simulink model "3-6-3"  (R2022b)
settings: Solver=VariableStepAuto  StartTime=0.0  StopTime=10.0  RelTol=1e-3
settings Model: Creator=Mavara-(Asus)  LastModifiedBy=Mavara-(Asus)

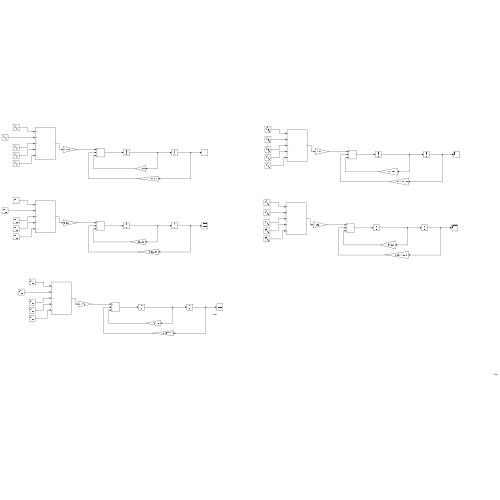
[thumbnail: Simulink's stored preview of the top-level diagram]
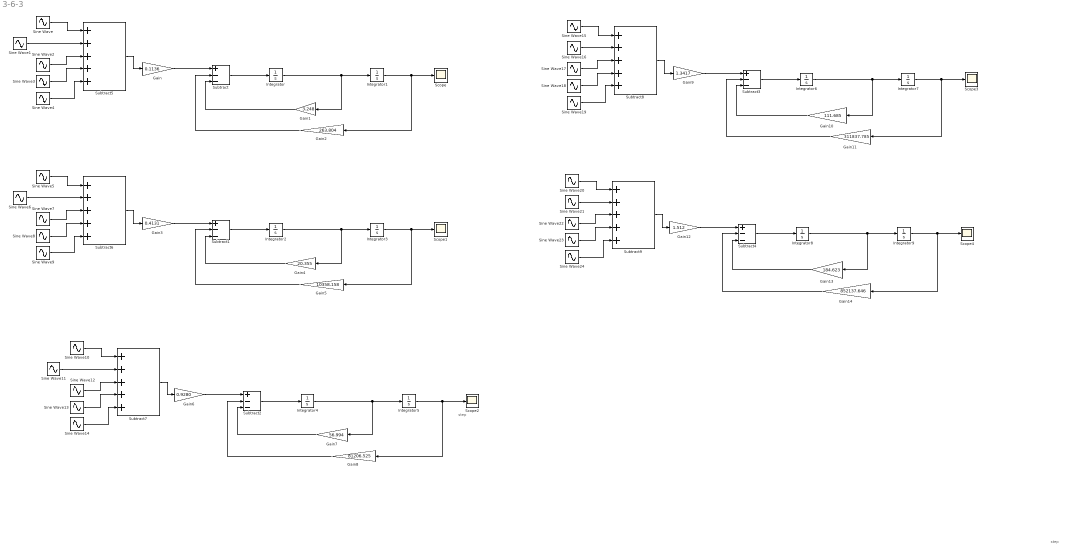
== system 3-6-3 ==
  note: step
  note: step
  Gain : Gain  Gain=0.1136
  Gain1 : Gain  Gain=3.248
  Gain10 : Gain  Gain=111.685
  Gain11 : Gain  Gain=311837.785
  Gain12 : Gain  Gain=1.512
  Gain13 : Gain  Gain=184.623
  Gain14 : Gain  Gain=852137.646
  Gain2 : Gain  Gain=263.804
  Gain3 : Gain  Gain=0.4131
  Gain4 : Gain  Gain=20.355
  Gain5 : Gain  Gain=10358.158
  Gain6 : Gain  Gain=0.9280
  Gain7 : Gain  Gain=56.994
  Gain8 : Gain  Gain=81206.525
  Gain9 : Gain  Gain=1.3417
  Integrator{,1..9} (10 alike) : Integrator
  Scope{,1..4} (5 alike) : Scope
  Sine Wave : Sin  Frequency=16.2338  SampleTime=0
  Sine Wave1 : Sin  Frequency=101.72344  SampleTime=0
  Sine Wave10 : Sin  Frequency=16.2338  SampleTime=0
  Sine Wave11 : Sin  Frequency=101.72344  SampleTime=0
  Sine Wave12 : Sin  Frequency=284.82312  SampleTime=0
  Sine Wave13 : Sin  Frequency=558.14128  SampleTime=0
  Sine Wave14 : Sin  Frequency=922.64504  SampleTime=0
  Sine Wave15 : Sin  Frequency=16.2338  SampleTime=0.01
  Sine Wave16 : Sin  Frequency=101.72344  SampleTime=0.01
  Sine Wave17 : Sin  Frequency=284.82312  SampleTime=0.01
  Sine Wave18 : Sin  Frequency=558.14128  SampleTime=0.01
  Sine Wave19 : Sin  Frequency=922.64504  SampleTime=0.01
  Sine Wave2 : Sin  Frequency=284.82312  SampleTime=0
  Sine Wave20 : Sin  Frequency=16.2338  SampleTime=0.1
  Sine Wave21 : Sin  Frequency=101.72344  SampleTime=0.1
  Sine Wave22 : Sin  Frequency=284.82312  SampleTime=0.1
  Sine Wave23 : Sin  Frequency=558.14128  SampleTime=0.1
  Sine Wave24 : Sin  Frequency=922.64504  SampleTime=0.1
  Sine Wave3 : Sin  Frequency=558.14128  SampleTime=0
  Sine Wave4 : Sin  Frequency=922.64504  SampleTime=0
  Sine Wave5 : Sin  Frequency=16.2338  SampleTime=0
  Sine Wave6 : Sin  Frequency=101.72344  SampleTime=0
  Sine Wave7 : Sin  Frequency=284.82312  SampleTime=0
  Sine Wave8 : Sin  Frequency=558.14128  SampleTime=0
  Sine Wave9 : Sin  Frequency=922.64504  SampleTime=0
  Subtract{,1..4} (5 alike) : Sum  Inputs=+--
  Subtract{5..9} (5 alike) : Sum  Inputs=+++++
  wires:
  Gain10/1 -> Subtract3/3
  Gain12/1 -> Subtract4/1
  Integrator7/1 -> Scope3/1, Gain11/1
  Integrator3/1 -> Scope1/1, Gain5/1
  Subtract4/1 -> Integrator8/1
  Gain11/1 -> Subtract3/2
  Gain9/1 -> Subtract3/1
  Gain7/1 -> Subtract2/3
  Integrator6/1 -> Gain10/1, Integrator7/1
  Gain14/1 -> Subtract4/2
  Gain1/1 -> Subtract/3
  Subtract2/1 -> Integrator4/1
  Integrator4/1 -> Gain7/1, Integrator5/1
  Integrator5/1 -> Scope2/1, Gain8/1
  Gain2/1 -> Subtract/2
  Gain6/1 -> Subtract2/1
  Integrator9/1 -> Scope4/1, Gain14/1
  Gain5/1 -> Subtract1/2
  Integrator8/1 -> Gain13/1, Integrator9/1
  Gain3/1 -> Subtract1/1
  Integrator2/1 -> Gain4/1, Integrator3/1
  Subtract3/1 -> Integrator6/1
  Integrator1/1 -> Scope/1, Gain2/1
  Integrator/1 -> Gain1/1, Integrator1/1
  Subtract/1 -> Integrator/1
  Subtract1/1 -> Integrator2/1
  Gain4/1 -> Subtract1/3
  Gain8/1 -> Subtract2/2
  Gain13/1 -> Subtract4/3
  Gain/1 -> Subtract/1
  Subtract5/1 -> Gain/1
  Sine Wave/1 -> Subtract5/1
  Sine Wave1/1 -> Subtract5/2
  Sine Wave2/1 -> Subtract5/3
  Sine Wave3/1 -> Subtract5/4
  Sine Wave4/1 -> Subtract5/5
  Sine Wave8/1 -> Subtract6/4
  Sine Wave9/1 -> Subtract6/5
  Sine Wave7/1 -> Subtract6/3
  Sine Wave5/1 -> Subtract6/1
  Subtract6/1 -> Gain3/1
  Sine Wave6/1 -> Subtract6/2
  Sine Wave13/1 -> Subtract7/4
  Sine Wave14/1 -> Subtract7/5
  Sine Wave12/1 -> Subtract7/3
  Sine Wave10/1 -> Subtract7/1
  Subtract7/1 -> Gain6/1
  Sine Wave11/1 -> Subtract7/2
  Sine Wave18/1 -> Subtract8/4
  Sine Wave19/1 -> Subtract8/5
  Sine Wave17/1 -> Subtract8/3
  Sine Wave15/1 -> Subtract8/1
  Subtract8/1 -> Gain9/1
  Sine Wave16/1 -> Subtract8/2
  Sine Wave23/1 -> Subtract9/4
  Sine Wave24/1 -> Subtract9/5
  Sine Wave22/1 -> Subtract9/3
  Sine Wave20/1 -> Subtract9/1
  Subtract9/1 -> Gain12/1
  Sine Wave21/1 -> Subtract9/2
